simulink model "model"  (R2020b)
settings: Solver=VariableStepAuto  StartTime=0.0  StopTime=(N-1)*Ts  RelTol=1e-3
model workspace (MATLAB code in the model file):
  | Gprocess = tf([-4 4],conv([6 1],[8 1]),'iodelay',2);
  | Ts = 0.8;
  | % Generate input signal
  | N = 2555;
  | u = idinput(N,'PRBS',[0 0.2],[-2 2]);
  | t = 0:Ts:Ts*(N-1);
  | input_moves = [t' u];
settings Model: Creator=HP  LastModifiedBy=HP

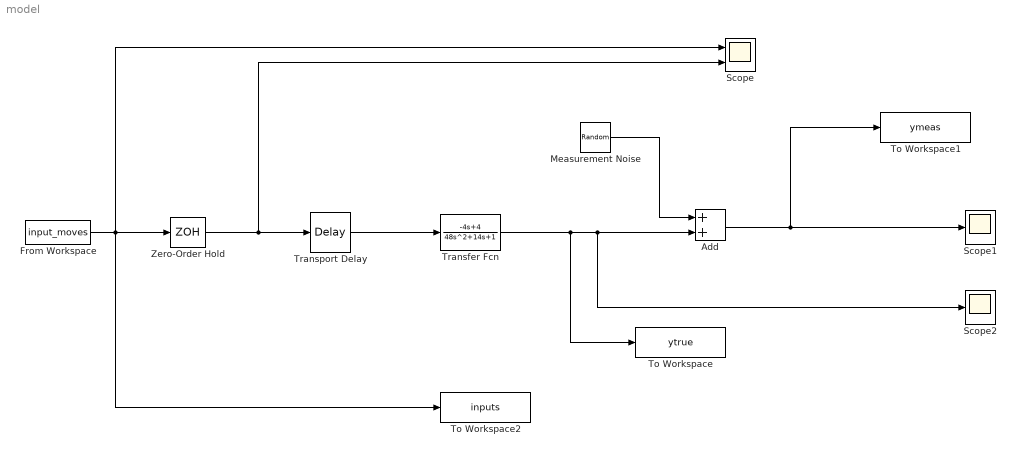
== system model ==
  Add : Sum
  From Workspace : FromWorkspace  VariableName=input_moves  SampleTime=Ts
  Measurement Noise : RandomNumber  Variance=1.2  SampleTime=Ts
  Scope : Scope  NumInputPorts=2
  Scope1 : Scope
  Scope2 : Scope
  To Workspace : ToWorkspace  VariableName=ytrue  SaveFormat=Timeseries  SampleTime=Ts
  To Workspace1 : ToWorkspace  VariableName=ymeas  SaveFormat=Timeseries  SampleTime=Ts
  To Workspace2 : ToWorkspace  VariableName=inputs  SaveFormat=Timeseries  SampleTime=Ts
  Transfer Fcn : TransferFcn  Numerator=[-4 4]  Denominator=[48 14 1]
  Transport Delay : TransportDelay  DelayTime=2
  Zero-Order Hold : ZeroOrderHold  SampleTime=Ts
  wires:
  Zero-Order Hold/1 -> Transport Delay/1, Scope/2
  Transfer Fcn/1 -> To Workspace/1, Scope2/1, Add/2
  From Workspace/1 -> To Workspace2/1, Scope/1, Zero-Order Hold/1
  Add/1 -> To Workspace1/1, Scope1/1
  Measurement Noise/1 -> Add/1
  Transport Delay/1 -> Transfer Fcn/1
